simulink model "Switched_Boost_Inverter_for_Standalone_system"  (R2020a)
settings: Solver=ode45  StartTime=0.0  StopTime=1.5  RelTol=1e-3  EnableMultiTasking=on
libraries: powerlib x24, simulink x9
settings Model: Creator=SONY  LastModifiedBy=sunil
settings DataIOCC: LimitDataPoints=on  SaveFormat=Array  SignalLoggingSaveFormat=ModelDataLogs  ReturnWorkspaceOutputs=off
settings OptimizationCC: LifeSpan=inf
settings DebuggingCC: UnderspecifiedInitializationDetection=Classic  MergeDetectMultiDrivingBlocksExec=none  SolverPrmCheckMsg=warning  FcnCallInpInsideContextMsg=warning  UnconnectedInputMsg=none  UnconnectedOutputMsg=none  UnconnectedLineMsg=none  StateNameClashWarn=warning  SFUnexpectedBacktrackingDiag=warning  SFNoUnconditionalDefaultTransitionDiag=warning  SFExecutionAtInitializationDiag=none  ArithmeticOperatorsInVariantConditions=warning
settings HardwareCC: ProdBitPerPointer=32  ProdBitPerSizeT=32  ProdBitPerPtrDiffT=32  ProdLargestAtomicFloat=None  ProdIntDivRoundTo=Undefined  ProdEndianess=Unspecified  ProdWordSize=32  ProdHWDeviceType=32-bit Generic
settings ModelReferenceCC: PropagateSignalLabelsOutOfModel=off
settings SFSimCC: SimUseLocalCustomCode=off  CustomCodeUndefinedFunction=UseInterfaceOnly
settings RTWCC: RTWUseLocalCustomCode=off
settings CodeAppCC: StateflowObjectComments=on
settings GRTTargetCC: TargetLangStandard=C89/C90 (ANSI)  CombineOutputUpdateFcns=off  GRTInterface=on
settings ConfigComp: CovMetricSettings=dw  CovHtmlReporting=on  CovSaveCumulativeToWorkspaceVar=on  CovSaveSingleToWorkspaceVar=on  CovExternalEMLEnable=off
settings SimscapeCC: SimscapeNormalizeSystem=off

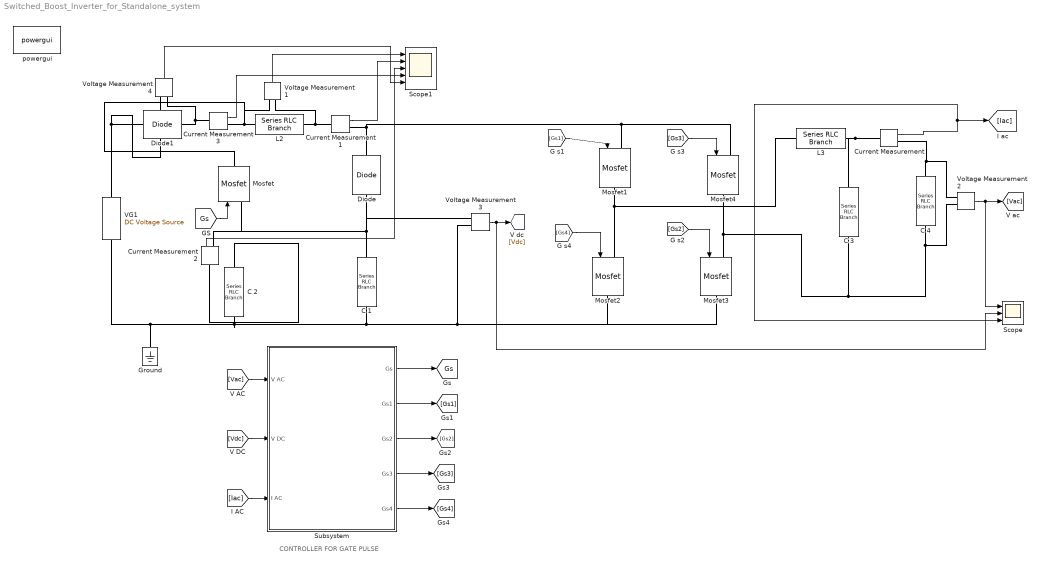
== system Switched_Boost_Inverter_for_Standalone_system ==
  note: CONTROLLER FOR GATE PULSE
  C 1 : powerlib/Elements/Series RLC Branch  LConnTagsString=__new0  RConnTagsString=__new0  BranchType=R  Resistance=70  Inductance=1e-3  SetiL0=off  InitialCurrent=0  Capacitance=1000e-6  Setx0=off  InitialVoltage=0  Measurements=None
  C 2 : powerlib/Elements/Series RLC Branch  LConnTagsString=__new0  RConnTagsString=__new0  BranchType=C  Resistance=1  Inductance=1e-3  SetiL0=off  InitialCurrent=0  Capacitance=10000e-6  Setx0=off  InitialVoltage=77  Measurements=None
  C 3 : powerlib/Elements/Series RLC Branch  LConnTagsString=__new0  RConnTagsString=__new0  BranchType=C  Resistance=1  Inductance=1e-3  SetiL0=off  InitialCurrent=0  Capacitance=.8e-3  Setx0=off  InitialVoltage=0  Measurements=None
  C 4 : powerlib/Elements/Series RLC Branch  LConnTagsString=__new0  RConnTagsString=__new0  BranchType=R  Resistance=210  Inductance=1e-3  SetiL0=off  InitialCurrent=0  Capacitance=1000e-6  Setx0=off  InitialVoltage=0  Measurements=None
  Current Measurement{,1..3} (4 alike) : powerlib/Measurements/Current Measurement  PhasorSimulation=off  OutputType=Complex  PSBequivalent=0
  Diode : powerlib/Power Electronics/Diode  Ron=0.001  Lon=0  Vf=0.8  IC=0  UseSnubber=off  Rs=inf  Cs=0  Measurements=off
  Diode1 : powerlib/Power Electronics/Diode  Ron=0.001  Lon=0  Vf=0.8  IC=0  UseSnubber=off  Rs=inf  Cs=0  Measurements=off
  Ground : powerlib/Elements/Ground  LConnTagsString=a
  L2 : powerlib/Elements/Series RLC Branch  LConnTagsString=__new0  RConnTagsString=__new0  BranchType=L  Resistance=0  Inductance=8500e-6  SetiL0=off  InitialCurrent=3  Capacitance=0  Setx0=off  InitialVoltage=0  Measurements=None
  L3 : powerlib/Elements/Series RLC Branch  LConnTagsString=__new0  RConnTagsString=__new0  BranchType=L  Resistance=0  Inductance=5e-3  SetiL0=off  InitialCurrent=0  Capacitance=0  Setx0=off  InitialVoltage=0  Measurements=None
  Mosfet{,1..4} (5 alike) : powerlib/Power Electronics/Mosfet  Ron=0.1  Lon=0  Rd=0.01  Vfd=0  IC=0  Rs=1e5  Cs=inf  Measurements=off
  Scope : Scope  NumInputPorts=3
  Scope1 : Scope  NumInputPorts=5
  Subsystem : Subsystem
  VG1 : powerlib/Electrical Sources/DC Voltage Source  Amplitude=48  Measurements=Voltage
  Voltage Measurement{1..4} (4 alike) : powerlib/Measurements/Voltage Measurement  PhasorSimulation=off  OutputType=Complex  PSBequivalent=0
  powergui : powerlib/powergui  Priority=1  SimulationMode=Discrete  SampleTime=50e-7  frequency=60  Iterations=50  frequencyindice=0  Pbase=100e6  ErrMax=1e-4  UnitsV=kV  UnitsW=MW  buscounter=0  FunctionMessages=off  echomessages=off  EnableUseOfTLC=off  CurrentSourceSwitches=off  DisableSnubberDevices=off  DisableRonSwitches=off  DisableVfSwitches=off  DisplayEquations=off  AutomaticDiscreteSolvers=off  SolverType=Tustin  Interpol=off  ExternalGateDelay=off  methode=off  Ts=0  x0status=blocks  SPID=off  SwTol=0  HookPort=off  NonlinearTolerance=1e-4  nMaxIteration=100  ContinueOnMaxIteration=off  RestoreLinks=warning  ResistiveCurrentMeasurement=off  Frange=[0:2:500]  Ylog=off  Xlog=on  ShowGrid=off  save=off  variable=ZData  structure=0  ZoomFFT=off  StartTime=0.0  cycles=1  DisplayStyle=1  fundamental=60  FreqAxis=off  MaxFrequency=1000  frequencyindicesteady=1  RmsSteady=1  display=off
  tag scope: Gs=global
  wires:
  Voltage Measurement3/1 -> Scope/2, [Vdc]
  [Gs1] -> Mosfet1/1
  [Gs4] -> Mosfet2/1
  [Gs2] -> Mosfet3/1
  Voltage Measurement2/1 -> Scope/1, [Vac]
  Subsystem/1(Gs) -> [Gs]
  Subsystem/2("Gs1 ") -> [Gs1]
  Subsystem/3(Gs2) -> [Gs2]
  Subsystem/4(Gs3) -> [Gs3]
  Subsystem/5(Gs4) -> [Gs4]
  [Vac] -> Subsystem/1(V AC)
  [Vdc] -> Subsystem/2(V DC)
  [Iac] -> Subsystem/3(I AC)
  [Gs3] -> Mosfet4/1
  Current Measurement/1 -> Scope/3, [Iac]
  Voltage Measurement1/1 -> Scope1/1
  Current Measurement1/1 -> Scope1/2
  Current Measurement2/1 -> Scope1/3
  Current Measurement3/1 -> Scope1/4
  Voltage Measurement4/1 -> Scope1/5
  [Gs] -> Mosfet/1
  connections:
  L3/LConn1 -- Mosfet2/LConn1 -- Mosfet1/RConn1
  Voltage Measurement2/LConn2 -- C 3/RConn1 -- Mosfet4/RConn1 -- Mosfet3/LConn1 -- C 4/LConn1
  VG1/LConn1 -- Ground/LConn1 -- C 1/LConn1 -- Voltage Measurement3/LConn2 -- Mosfet3/RConn1 -- Mosfet2/RConn1 -- C 2/RConn1
  C 4/RConn1 -- Current Measurement/RConn1 -- Voltage Measurement2/LConn1
  Current Measurement/LConn1 -- C 3/LConn1 -- L3/RConn1
  VG1/RConn1 -- Voltage Measurement4/LConn1 -- Diode1/LConn1
  Voltage Measurement3/LConn1 -- Diode/RConn1 -- Current Measurement2/RConn1 -- Mosfet/LConn1 -- C 1/RConn1
  Mosfet4/LConn1 -- Current Measurement1/RConn1 -- Diode/LConn1 -- Mosfet1/LConn1
  Current Measurement3/RConn1 -- Mosfet/RConn1 -- Voltage Measurement1/LConn1 -- L2/LConn1
  Current Measurement1/LConn1 -- Voltage Measurement1/LConn2 -- L2/RConn1
  C 2/LConn1 -- Current Measurement2/LConn1
  Current Measurement3/LConn1 -- Voltage Measurement4/LConn2 -- Diode1/RConn1

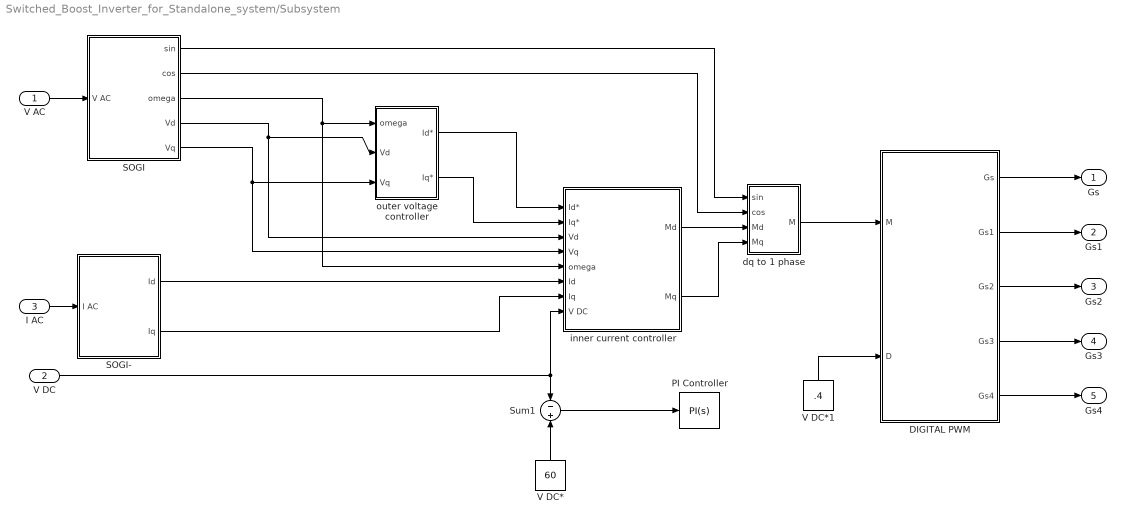
== system Switched_Boost_Inverter_for_Standalone_system/Subsystem ==
  V AC : Inport
  V DC : Inport  Port=2
  I AC : Inport  Port=3
  DIGITAL PWM : Subsystem
  PI Controller : simulink/Continuous/PID Controller  Controller=PI  Form=Parallel  TimeDomain=Continuous-time  UseExternalTs=off  SampleTime=1  IntegratorMethod=Forward Euler  FilterMethod=Forward Euler  ControllerParametersSource=internal  P=.0001  I=1  D=-0.695594942304429  UseFilter=on  N=5248.00493874348  TunerSelectOption=Transfer Function Based (PID Tuner App)  InitialConditionSource=internal  InitialConditionForIntegrator=0  InitialConditionForFilter=0  DifferentiatorICPrevScaledInput=0  ExternalReset=none  TrackingMode=off  Kt=1  LimitOutput=off  UpperSaturationLimit=inf  LowerSaturationLimit=-inf  LinearizeAsGain=off  AntiWindupMode=none  Kb=1  POutMin=[]  POutMax=[]  IOutMin=[]  IOutMax=[]  DOutMin=[]  DOutMax=[]  NOutMin=[]  NOutMax=[]  SumOutMin=[]  SumOutMax=[]  SaturationOutMin=[]  SaturationOutMax=[]  PParamMin=[]  PParamMax=[]  IParamMin=[]  IParamMax=[]  DParamMin=[]  DParamMax=[]  NParamMin=[]  NParamMax=[]  KbParamMin=[]  KbParamMax=[]  KtParamMin=[]  KtParamMax=[]  KbOutMin=[]  KbOutMax=[]  KtOutMin=[]  KtOutMax=[]  IntegratorOutMin=[]  IntegratorOutMax=[]  FilterOutMin=[]  FilterOutMax=[]  SumI1OutMin=[]  SumI1OutMax=[]  SumI2OutMin=[]  SumI2OutMax=[]  SumI3OutMin=[]  SumI3OutMax=[]  SumI4OutMin=[]  SumI4OutMax=[]  SumDOutMin=[]  SumDOutMax=[]  DifferentiatorOutMin=[]  DifferentiatorOutMax=[]  FilterDiffOutCoefMin=[]  FilterDiffOutCoefMax=[]  ReciprocalOutMin=[]  ReciprocalOutMax=[]  SumDenOutMin=[]  SumDenOutMax=[]  SumNumOutMin=[]  SumNumOutMax=[]  DivideOutMin=[]  DivideOutMax=[]  UdiffTsProdOutMin=[]  UdiffTsProdOutMax=[]  NTsProdOutMin=[]  NTsProdOutMax=[]  UintegralTsProdOutMin=[]  UintegralTsProdOutMax=[]  UngainTsProdOutMin=[]  UngainTsProdOutMax=[]  IntegratorContinuousStateAttributes=''  IntegratorStateMustResolveToSignalObject=off  IntegratorRTWStateStorageClass=Auto  FilterContinuousStateAttributes=''  FilterStateMustResolveToSignalObject=off  FilterRTWStateStorageClass=Auto  ParallelPVariant=InternalParameters  IdealPVariant=Disabled  IVariant=InternalParameters  DVariant=Disabled  IntegratorVariant=Continuous  SatVariant=Disabled  AWVariant=Passthrough  PCopyVariant=Disabled  TRVariant=Disabled  FdbkBlocksVariant=Forward  IdealPFdbkVariant=Disabled  SatFdbkVariant=Disabled  DerivativeFilterVariant=Disabled  NVariant=Disabled  NCopyVariant=Disabled_SignalSpec  FilterICVariant=Disabled  IntegratorICVariant=InternalICs  ExternalResetVariant=Disabled  TRSumVariant=Passthrough  SumFdbkVariant=Disabled  SumVariant=Sum_PI  TsampFilterVariant=InternalTs  TsampNgainVariant=Passthrough  TsampIntegralVariant=Passthrough
  SOGI : Subsystem
  SOGI- : Subsystem
  Sum1 : Sum  Inputs=-+
  V DC* : Constant  Value=60
  V DC*1 : Constant  Value=.4
  dq to 1 phase : Subsystem
  inner current controller : Subsystem
  outer voltage controller : Subsystem
  Gs : Outport  InitialOutput=0
  "Gs1 " : Outport  Port=2  InitialOutput=0
  Gs2 : Outport  Port=3  InitialOutput=0
  Gs3 : Outport  Port=4  InitialOutput=0
  Gs4 : Outport  Port=5  InitialOutput=0
  wires:
  V AC/1 -> SOGI/1(V AC)
  I AC/1 -> SOGI-/1(I AC)
  SOGI/4(Vd) -> inner current controller/3(Vd), outer voltage controller/2(Vd)
  SOGI/5(Vq) -> inner current controller/4(Vq), outer voltage controller/3(Vq)
  SOGI-/1(Id) -> inner current controller/6(Id)
  SOGI-/2(Iq) -> inner current controller/7(Iq)
  V DC/1 -> inner current controller/8(V DC), Sum1/1
  outer voltage controller/1(Id*) -> inner current controller/1(Id*)
  outer voltage controller/2(Iq*) -> inner current controller/2(Iq*)
  Sum1/1 -> PI Controller/1
  V DC*/1 -> Sum1/2
  inner current controller/1(Md) -> dq to 1 phase/3(Md)
  inner current controller/2(Mq) -> dq to 1 phase/4(Mq)
  DIGITAL PWM/1(Gs) -> Gs/1
  DIGITAL PWM/2("Gs1 ") -> "Gs1 "/1
  DIGITAL PWM/3(Gs2) -> Gs2/1
  DIGITAL PWM/4(Gs3) -> Gs3/1
  DIGITAL PWM/5(Gs4) -> Gs4/1
  SOGI/3(omega) -> inner current controller/5(omega), outer voltage controller/1(omega)
  SOGI/1(sin) -> dq to 1 phase/1(sin)
  SOGI/2(cos) -> dq to 1 phase/2(cos)
  V DC*1/1 -> DIGITAL PWM/2(D)
  dq to 1 phase/1(M) -> DIGITAL PWM/1(M)

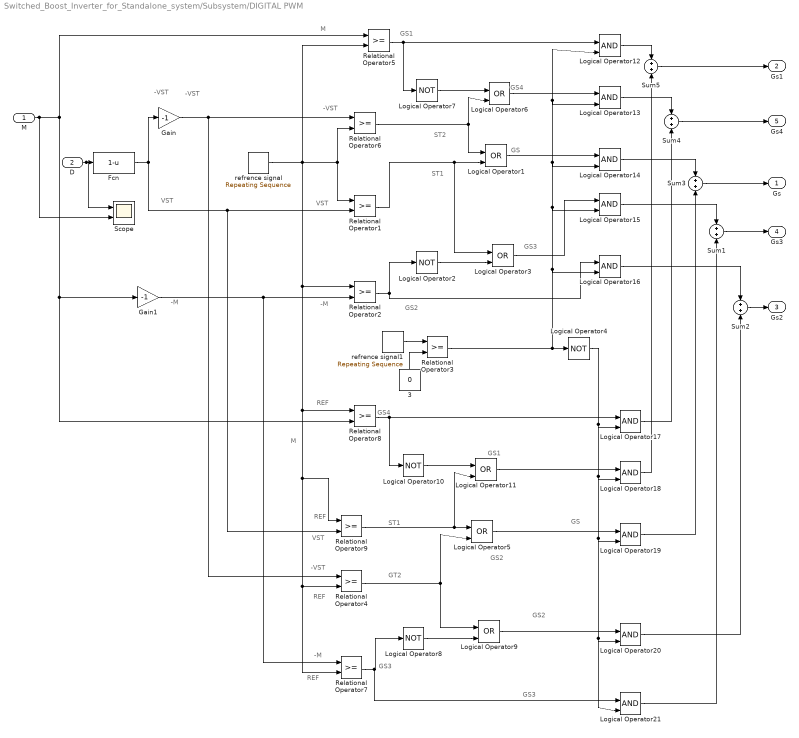
== system Switched_Boost_Inverter_for_Standalone_system/Subsystem/DIGITAL PWM ==
  note: GS3
  note: GS2
  note: GS
  note: GS2
  note: GS3
  note: GS
  note: GS4
  note: GS1
  note: -M
  note: VST
  note: -VST
  note: M
  note: GT2
  note: ST1
  note: -M
  note: -VST
  note: VST
  note: REF
  note: REF
  note: REF
  note: REF
  note: VST
  note: -VST
  note: -VST
  note: -M
  note: GS3
  note: GS2
  note: GS1
  note: GS4
  note: ST1
  note: ST2
  note: M
  M : Inport
  D : Inport  Port=2
  3 : Constant  Value=0
  Fcn : Fcn  Expr=1-u
  Gain : Gain  Gain=-1
  Gain1 : Gain  Gain=-1
  Logical Operator{1,3,5..6,9,11} (6 alike) : Logic  Operator=OR  IconShape=distinctive  AllPortsSameDT=off  OutDataTypeStr=boolean
  Logical Operator{2,4,7..8,10} (5 alike) : Logic  Operator=NOT  IconShape=distinctive  AllPortsSameDT=off  OutDataTypeStr=boolean
  Logical Operator{12..21} (10 alike) : Logic  IconShape=distinctive  AllPortsSameDT=off  OutDataTypeStr=boolean
  Relational Operator{1..9} (9 alike) : RelationalOperator  OutDataTypeStr=boolean  RndMeth=Nearest
  Scope : Scope  NumInputPorts=2
  Sum{1..5} (5 alike) : Sum
  refrence signal : simulink/Sources/Repeating Sequence  rep_seq_t="[0 .00005  .0001]"  rep_seq_y="[1 -1  1 ]"
  refrence signal1 : simulink/Sources/Repeating Sequence  rep_seq_t="[0  .01  .02]"  rep_seq_y="[1  0  -1  ]"
  Gs : Outport  InitialOutput=0
  "Gs1 " : Outport  Port=2  InitialOutput=0
  Gs2 : Outport  Port=3  InitialOutput=0
  Gs3 : Outport  Port=4  InitialOutput=0
  Gs4 : Outport  Port=5  InitialOutput=0
  wires:
  Gain/1 -> Relational Operator4/1, Relational Operator6/1
  Relational Operator5/1 -> Logical Operator7/1, Logical Operator12/1
  Logical Operator7/1 -> Logical Operator6/1
  Relational Operator6/1 -> Logical Operator1/1, Logical Operator6/2
  Relational Operator1/1 -> Logical Operator1/2, Logical Operator3/1
  Gain1/1 -> Relational Operator7/1, Relational Operator2/2
  Relational Operator2/1 -> Logical Operator2/1, Logical Operator16/1
  Logical Operator2/1 -> Logical Operator3/2
  D/1 -> Scope/1, Fcn/1
  Relational Operator8/1 -> Logical Operator17/1, Logical Operator10/1
  Logical Operator10/1 -> Logical Operator11/1
  Relational Operator9/1 -> Logical Operator11/2, Logical Operator5/1
  Relational Operator4/1 -> Logical Operator5/2, Logical Operator9/1
  Relational Operator7/1 -> Logical Operator21/1, Logical Operator8/1
  Logical Operator8/1 -> Logical Operator9/2
  Fcn/1 -> Relational Operator9/2, Relational Operator1/2, Gain/1
  refrence signal/1 -> Relational Operator8/1, Relational Operator9/1, Relational Operator4/2, Relational Operator7/2, Relational Operator2/1, Relational Operator5/2, Relational Operator1/1, Relational Operator6/2
  M/1 -> Scope/2, Relational Operator5/1, Relational Operator8/2, Gain1/1
  refrence signal1/1 -> Relational Operator3/1
  3/1 -> Relational Operator3/2
  Logical Operator4/1 -> Logical Operator20/2, Logical Operator21/2, Logical Operator19/2, Logical Operator18/2, Logical Operator17/2
  Logical Operator6/1 -> Logical Operator13/1
  Logical Operator1/1 -> Logical Operator14/1
  Logical Operator3/1 -> Logical Operator15/1
  Relational Operator3/1 -> Logical Operator16/2, Logical Operator15/2, Logical Operator14/2, Logical Operator13/2, Logical Operator12/2, Logical Operator4/1
  Logical Operator11/1 -> Logical Operator18/1
  Logical Operator5/1 -> Logical Operator19/1
  Logical Operator9/1 -> Logical Operator20/1
  Logical Operator12/1 -> Sum5/1
  Sum5/1 -> "Gs1 "/1
  Logical Operator18/1 -> Sum5/2
  Logical Operator13/1 -> Sum4/1
  Sum4/1 -> Gs4/1
  Logical Operator17/1 -> Sum4/2
  Logical Operator14/1 -> Sum3/1
  Sum3/1 -> Gs/1
  Logical Operator19/1 -> Sum3/2
  Logical Operator16/1 -> Sum2/1
  Logical Operator15/1 -> Sum1/1
  Sum1/1 -> Gs3/1
  Logical Operator21/1 -> Sum1/2
  Sum2/1 -> Gs2/1
  Logical Operator20/1 -> Sum2/2

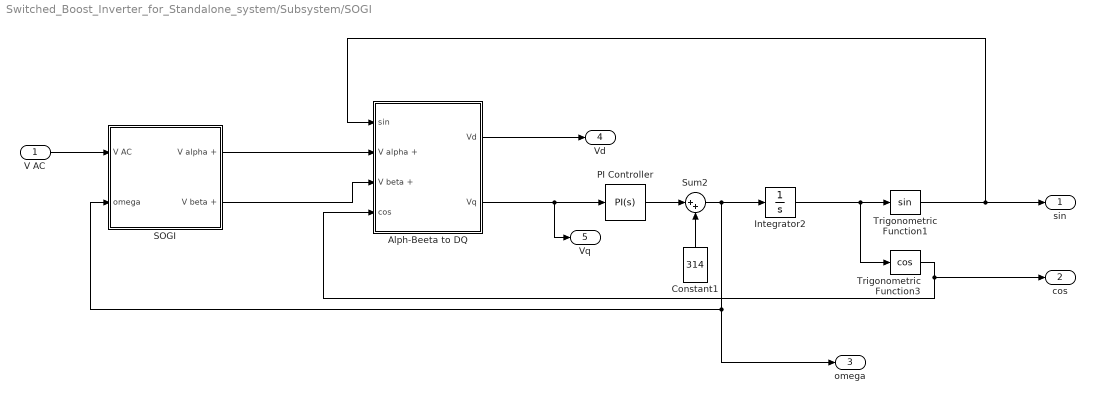
== system Switched_Boost_Inverter_for_Standalone_system/Subsystem/SOGI ==
  V AC : Inport
  Alph-Beeta to DQ : Subsystem
  Constant1 : Constant  Value=314
  Integrator2 : Integrator
  PI Controller : simulink/Continuous/PID Controller  Controller=PI  Form=Parallel  TimeDomain=Continuous-time  UseExternalTs=off  SampleTime=1  IntegratorMethod=Forward Euler  FilterMethod=Forward Euler  ControllerParametersSource=internal  P=1  I=2  D=-0.695594942304429  UseFilter=on  N=5248.00493874348  TunerSelectOption=Transfer Function Based (PID Tuner App)  InitialConditionSource=internal  InitialConditionForIntegrator=0  InitialConditionForFilter=0  DifferentiatorICPrevScaledInput=0  ExternalReset=none  TrackingMode=off  Kt=1  LimitOutput=off  UpperSaturationLimit=inf  LowerSaturationLimit=-inf  LinearizeAsGain=off  AntiWindupMode=none  Kb=1  POutMin=[]  POutMax=[]  IOutMin=[]  IOutMax=[]  DOutMin=[]  DOutMax=[]  NOutMin=[]  NOutMax=[]  SumOutMin=[]  SumOutMax=[]  SaturationOutMin=[]  SaturationOutMax=[]  PParamMin=[]  PParamMax=[]  IParamMin=[]  IParamMax=[]  DParamMin=[]  DParamMax=[]  NParamMin=[]  NParamMax=[]  KbParamMin=[]  KbParamMax=[]  KtParamMin=[]  KtParamMax=[]  KbOutMin=[]  KbOutMax=[]  KtOutMin=[]  KtOutMax=[]  IntegratorOutMin=[]  IntegratorOutMax=[]  FilterOutMin=[]  FilterOutMax=[]  SumI1OutMin=[]  SumI1OutMax=[]  SumI2OutMin=[]  SumI2OutMax=[]  SumI3OutMin=[]  SumI3OutMax=[]  SumI4OutMin=[]  SumI4OutMax=[]  SumDOutMin=[]  SumDOutMax=[]  DifferentiatorOutMin=[]  DifferentiatorOutMax=[]  FilterDiffOutCoefMin=[]  FilterDiffOutCoefMax=[]  ReciprocalOutMin=[]  ReciprocalOutMax=[]  SumDenOutMin=[]  SumDenOutMax=[]  SumNumOutMin=[]  SumNumOutMax=[]  DivideOutMin=[]  DivideOutMax=[]  UdiffTsProdOutMin=[]  UdiffTsProdOutMax=[]  NTsProdOutMin=[]  NTsProdOutMax=[]  UintegralTsProdOutMin=[]  UintegralTsProdOutMax=[]  UngainTsProdOutMin=[]  UngainTsProdOutMax=[]  IntegratorContinuousStateAttributes=''  IntegratorStateMustResolveToSignalObject=off  IntegratorRTWStateStorageClass=Auto  FilterContinuousStateAttributes=''  FilterStateMustResolveToSignalObject=off  FilterRTWStateStorageClass=Auto  ParallelPVariant=InternalParameters  IdealPVariant=Disabled  IVariant=InternalParameters  DVariant=Disabled  IntegratorVariant=Continuous  SatVariant=Disabled  AWVariant=Passthrough  PCopyVariant=Disabled  TRVariant=Disabled  FdbkBlocksVariant=Forward  IdealPFdbkVariant=Disabled  SatFdbkVariant=Disabled  DerivativeFilterVariant=Disabled  NVariant=Disabled  NCopyVariant=Disabled_SignalSpec  FilterICVariant=Disabled  IntegratorICVariant=InternalICs  ExternalResetVariant=Disabled  TRSumVariant=Passthrough  SumFdbkVariant=Disabled  SumVariant=Sum_PI  TsampFilterVariant=InternalTs  TsampNgainVariant=Passthrough  TsampIntegralVariant=Passthrough
  SOGI : Subsystem
  Sum2 : Sum  Inputs=|++
  Trigonometric Function1 : Trigonometry
  Trigonometric Function3 : Trigonometry  Operator=cos
  sin : Outport
  cos : Outport  Port=2
  omega : Outport  Port=3
  Vd : Outport  Port=4
  Vq : Outport  Port=5
  wires:
  Sum2/1 -> omega/1, SOGI/2(omega), Integrator2/1
  SOGI/1(V alpha +) -> Alph-Beeta to DQ/2(V alpha +)
  SOGI/2(V beta +) -> Alph-Beeta to DQ/3(V beta +)
  Trigonometric Function3/1 -> cos/1, Alph-Beeta to DQ/4(cos)
  Integrator2/1 -> Trigonometric Function3/1, Trigonometric Function1/1
  Alph-Beeta to DQ/1(Vd) -> Vd/1
  PI Controller/1 -> Sum2/1
  Constant1/1 -> Sum2/2
  Trigonometric Function1/1 -> Alph-Beeta to DQ/1(sin), sin/1
  Alph-Beeta to DQ/2(Vq) -> PI Controller/1, Vq/1
  V AC/1 -> SOGI/1(V AC)

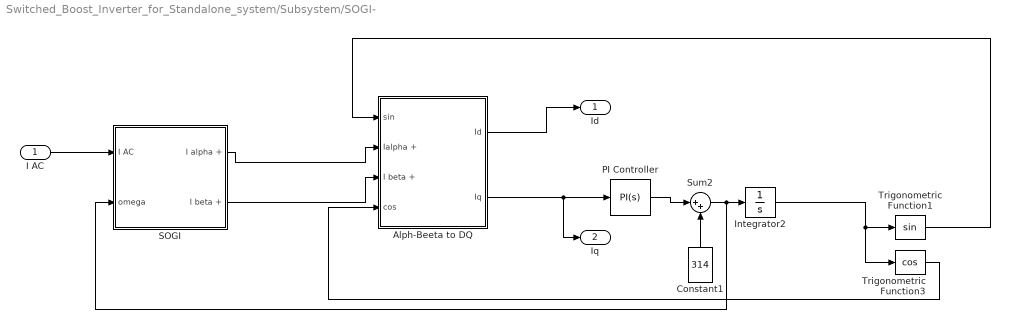
== system Switched_Boost_Inverter_for_Standalone_system/Subsystem/SOGI- ==
  I AC : Inport
  Alph-Beeta to DQ : Subsystem
  Constant1 : Constant  Value=314
  Integrator2 : Integrator
  PI Controller : simulink/Continuous/PID Controller  Controller=PI  Form=Parallel  TimeDomain=Continuous-time  UseExternalTs=off  SampleTime=1  IntegratorMethod=Forward Euler  FilterMethod=Forward Euler  ControllerParametersSource=internal  P=1  I=2  D=-0.695594942304429  UseFilter=on  N=5248.00493874348  TunerSelectOption=Transfer Function Based (PID Tuner App)  InitialConditionSource=internal  InitialConditionForIntegrator=0  InitialConditionForFilter=0  DifferentiatorICPrevScaledInput=0  ExternalReset=none  TrackingMode=off  Kt=1  LimitOutput=off  UpperSaturationLimit=inf  LowerSaturationLimit=-inf  LinearizeAsGain=off  AntiWindupMode=none  Kb=1  POutMin=[]  POutMax=[]  IOutMin=[]  IOutMax=[]  DOutMin=[]  DOutMax=[]  NOutMin=[]  NOutMax=[]  SumOutMin=[]  SumOutMax=[]  SaturationOutMin=[]  SaturationOutMax=[]  PParamMin=[]  PParamMax=[]  IParamMin=[]  IParamMax=[]  DParamMin=[]  DParamMax=[]  NParamMin=[]  NParamMax=[]  KbParamMin=[]  KbParamMax=[]  KtParamMin=[]  KtParamMax=[]  KbOutMin=[]  KbOutMax=[]  KtOutMin=[]  KtOutMax=[]  IntegratorOutMin=[]  IntegratorOutMax=[]  FilterOutMin=[]  FilterOutMax=[]  SumI1OutMin=[]  SumI1OutMax=[]  SumI2OutMin=[]  SumI2OutMax=[]  SumI3OutMin=[]  SumI3OutMax=[]  SumI4OutMin=[]  SumI4OutMax=[]  SumDOutMin=[]  SumDOutMax=[]  DifferentiatorOutMin=[]  DifferentiatorOutMax=[]  FilterDiffOutCoefMin=[]  FilterDiffOutCoefMax=[]  ReciprocalOutMin=[]  ReciprocalOutMax=[]  SumDenOutMin=[]  SumDenOutMax=[]  SumNumOutMin=[]  SumNumOutMax=[]  DivideOutMin=[]  DivideOutMax=[]  UdiffTsProdOutMin=[]  UdiffTsProdOutMax=[]  NTsProdOutMin=[]  NTsProdOutMax=[]  UintegralTsProdOutMin=[]  UintegralTsProdOutMax=[]  UngainTsProdOutMin=[]  UngainTsProdOutMax=[]  IntegratorContinuousStateAttributes=''  IntegratorStateMustResolveToSignalObject=off  IntegratorRTWStateStorageClass=Auto  FilterContinuousStateAttributes=''  FilterStateMustResolveToSignalObject=off  FilterRTWStateStorageClass=Auto  ParallelPVariant=InternalParameters  IdealPVariant=Disabled  IVariant=InternalParameters  DVariant=Disabled  IntegratorVariant=Continuous  SatVariant=Disabled  AWVariant=Passthrough  PCopyVariant=Disabled  TRVariant=Disabled  FdbkBlocksVariant=Forward  IdealPFdbkVariant=Disabled  SatFdbkVariant=Disabled  DerivativeFilterVariant=Disabled  NVariant=Disabled  NCopyVariant=Disabled_SignalSpec  FilterICVariant=Disabled  IntegratorICVariant=InternalICs  ExternalResetVariant=Disabled  TRSumVariant=Passthrough  SumFdbkVariant=Disabled  SumVariant=Sum_PI  TsampFilterVariant=InternalTs  TsampNgainVariant=Passthrough  TsampIntegralVariant=Passthrough
  SOGI : Subsystem
  Sum2 : Sum  Inputs=|++
  Trigonometric Function1 : Trigonometry
  Trigonometric Function3 : Trigonometry  Operator=cos
  Id : Outport
  Iq : Outport  Port=2
  wires:
  Sum2/1 -> SOGI/2(omega), Integrator2/1
  SOGI/1(I alpha +) -> Alph-Beeta to DQ/2(Ialpha +)
  SOGI/2(I beta +) -> Alph-Beeta to DQ/3(I beta +)
  Trigonometric Function3/1 -> Alph-Beeta to DQ/4(cos)
  Integrator2/1 -> Trigonometric Function1/1, Trigonometric Function3/1
  Alph-Beeta to DQ/1(Id) -> Id/1
  PI Controller/1 -> Sum2/1
  Constant1/1 -> Sum2/2
  Trigonometric Function1/1 -> Alph-Beeta to DQ/1(sin)
  Alph-Beeta to DQ/2(Iq) -> Iq/1, PI Controller/1
  I AC/1 -> SOGI/1(I AC)

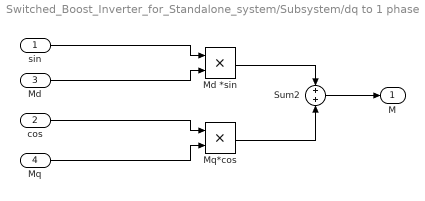
== system Switched_Boost_Inverter_for_Standalone_system/Subsystem/dq to 1 phase ==
  sin : Inport
  cos : Inport  Port=2
  Md : Inport  Port=3
  Mq : Inport  Port=4
  Md *sin : Product  Inputs=**
  Mq*cos : Product  Inputs=**
  Sum2 : Sum
  M : Outport  InitialOutput=0
  wires:
  Md/1 -> Md *sin/2
  cos/1 -> Mq*cos/1
  Mq*cos/1 -> Sum2/2
  Sum2/1 -> M/1
  Mq/1 -> Mq*cos/2
  Md *sin/1 -> Sum2/1
  sin/1 -> Md *sin/1

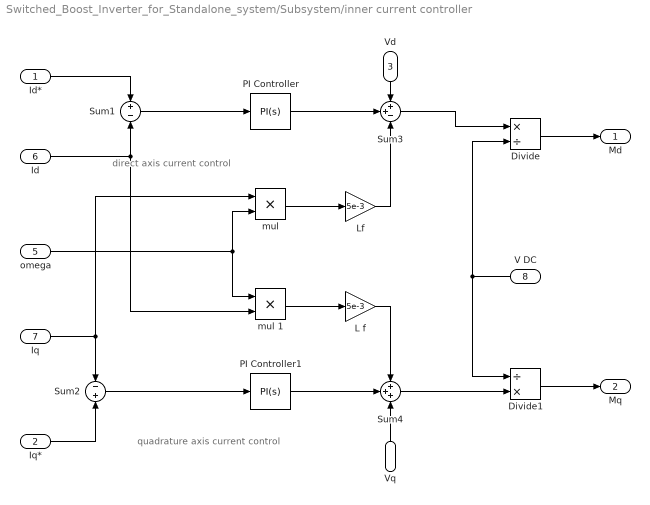
== system Switched_Boost_Inverter_for_Standalone_system/Subsystem/inner current controller ==
  note: quadrature axis current control
  note: direct axis current control
  Id* : Inport
  Iq* : Inport  Port=2
  Vd : Inport  Port=3
  Vq : Inport  Port=4
  omega : Inport  Port=5
  Id : Inport  Port=6
  Iq : Inport  Port=7
  V DC : Inport  Port=8
  Divide : Product  Inputs=*/
  Divide1 : Product  Inputs=/*
  L f : Gain  Gain=5e-3
  Lf : Gain  Gain=5e-3
  PI Controller : simulink/Continuous/PID Controller  Controller=PI  Form=Parallel  TimeDomain=Continuous-time  UseExternalTs=off  SampleTime=1  IntegratorMethod=Forward Euler  FilterMethod=Forward Euler  ControllerParametersSource=internal  P=.01  I=.09  D=-0.695594942304429  UseFilter=on  N=5248.00493874348  TunerSelectOption=Transfer Function Based (PID Tuner App)  InitialConditionSource=internal  InitialConditionForIntegrator=0  InitialConditionForFilter=0  DifferentiatorICPrevScaledInput=0  ExternalReset=none  TrackingMode=off  Kt=1  LimitOutput=off  UpperSaturationLimit=inf  LowerSaturationLimit=-inf  LinearizeAsGain=off  AntiWindupMode=none  Kb=1  POutMin=[]  POutMax=[]  IOutMin=[]  IOutMax=[]  DOutMin=[]  DOutMax=[]  NOutMin=[]  NOutMax=[]  SumOutMin=[]  SumOutMax=[]  SaturationOutMin=[]  SaturationOutMax=[]  PParamMin=[]  PParamMax=[]  IParamMin=[]  IParamMax=[]  DParamMin=[]  DParamMax=[]  NParamMin=[]  NParamMax=[]  KbParamMin=[]  KbParamMax=[]  KtParamMin=[]  KtParamMax=[]  KbOutMin=[]  KbOutMax=[]  KtOutMin=[]  KtOutMax=[]  IntegratorOutMin=[]  IntegratorOutMax=[]  FilterOutMin=[]  FilterOutMax=[]  SumI1OutMin=[]  SumI1OutMax=[]  SumI2OutMin=[]  SumI2OutMax=[]  SumI3OutMin=[]  SumI3OutMax=[]  SumI4OutMin=[]  SumI4OutMax=[]  SumDOutMin=[]  SumDOutMax=[]  DifferentiatorOutMin=[]  DifferentiatorOutMax=[]  FilterDiffOutCoefMin=[]  FilterDiffOutCoefMax=[]  ReciprocalOutMin=[]  ReciprocalOutMax=[]  SumDenOutMin=[]  SumDenOutMax=[]  SumNumOutMin=[]  SumNumOutMax=[]  DivideOutMin=[]  DivideOutMax=[]  UdiffTsProdOutMin=[]  UdiffTsProdOutMax=[]  NTsProdOutMin=[]  NTsProdOutMax=[]  UintegralTsProdOutMin=[]  UintegralTsProdOutMax=[]  UngainTsProdOutMin=[]  UngainTsProdOutMax=[]  IntegratorContinuousStateAttributes=''  IntegratorStateMustResolveToSignalObject=off  IntegratorRTWStateStorageClass=Auto  FilterContinuousStateAttributes=''  FilterStateMustResolveToSignalObject=off  FilterRTWStateStorageClass=Auto  ParallelPVariant=InternalParameters  IdealPVariant=Disabled  IVariant=InternalParameters  DVariant=Disabled  IntegratorVariant=Continuous  SatVariant=Disabled  AWVariant=Passthrough  PCopyVariant=Disabled  TRVariant=Disabled  FdbkBlocksVariant=Forward  IdealPFdbkVariant=Disabled  SatFdbkVariant=Disabled  DerivativeFilterVariant=Disabled  NVariant=Disabled  NCopyVariant=Disabled_SignalSpec  FilterICVariant=Disabled  IntegratorICVariant=InternalICs  ExternalResetVariant=Disabled  TRSumVariant=Passthrough  SumFdbkVariant=Disabled  SumVariant=Sum_PI  TsampFilterVariant=InternalTs  TsampNgainVariant=Passthrough  TsampIntegralVariant=Passthrough
  PI Controller1 : simulink/Continuous/PID Controller  Controller=PI  Form=Parallel  TimeDomain=Continuous-time  UseExternalTs=off  SampleTime=1  IntegratorMethod=Forward Euler  FilterMethod=Forward Euler  ControllerParametersSource=internal  P=.01  I=.09  D=-0.695594942304429  UseFilter=on  N=5248.00493874348  TunerSelectOption=Transfer Function Based (PID Tuner App)  InitialConditionSource=internal  InitialConditionForIntegrator=0  InitialConditionForFilter=0  DifferentiatorICPrevScaledInput=0  ExternalReset=none  TrackingMode=off  Kt=1  LimitOutput=off  UpperSaturationLimit=inf  LowerSaturationLimit=-inf  LinearizeAsGain=off  AntiWindupMode=none  Kb=1  POutMin=[]  POutMax=[]  IOutMin=[]  IOutMax=[]  DOutMin=[]  DOutMax=[]  NOutMin=[]  NOutMax=[]  SumOutMin=[]  SumOutMax=[]  SaturationOutMin=[]  SaturationOutMax=[]  PParamMin=[]  PParamMax=[]  IParamMin=[]  IParamMax=[]  DParamMin=[]  DParamMax=[]  NParamMin=[]  NParamMax=[]  KbParamMin=[]  KbParamMax=[]  KtParamMin=[]  KtParamMax=[]  KbOutMin=[]  KbOutMax=[]  KtOutMin=[]  KtOutMax=[]  IntegratorOutMin=[]  IntegratorOutMax=[]  FilterOutMin=[]  FilterOutMax=[]  SumI1OutMin=[]  SumI1OutMax=[]  SumI2OutMin=[]  SumI2OutMax=[]  SumI3OutMin=[]  SumI3OutMax=[]  SumI4OutMin=[]  SumI4OutMax=[]  SumDOutMin=[]  SumDOutMax=[]  DifferentiatorOutMin=[]  DifferentiatorOutMax=[]  FilterDiffOutCoefMin=[]  FilterDiffOutCoefMax=[]  ReciprocalOutMin=[]  ReciprocalOutMax=[]  SumDenOutMin=[]  SumDenOutMax=[]  SumNumOutMin=[]  SumNumOutMax=[]  DivideOutMin=[]  DivideOutMax=[]  UdiffTsProdOutMin=[]  UdiffTsProdOutMax=[]  NTsProdOutMin=[]  NTsProdOutMax=[]  UintegralTsProdOutMin=[]  UintegralTsProdOutMax=[]  UngainTsProdOutMin=[]  UngainTsProdOutMax=[]  IntegratorContinuousStateAttributes=''  IntegratorStateMustResolveToSignalObject=off  IntegratorRTWStateStorageClass=Auto  FilterContinuousStateAttributes=''  FilterStateMustResolveToSignalObject=off  FilterRTWStateStorageClass=Auto  ParallelPVariant=InternalParameters  IdealPVariant=Disabled  IVariant=InternalParameters  DVariant=Disabled  IntegratorVariant=Continuous  SatVariant=Disabled  AWVariant=Passthrough  PCopyVariant=Disabled  TRVariant=Disabled  FdbkBlocksVariant=Forward  IdealPFdbkVariant=Disabled  SatFdbkVariant=Disabled  DerivativeFilterVariant=Disabled  NVariant=Disabled  NCopyVariant=Disabled_SignalSpec  FilterICVariant=Disabled  IntegratorICVariant=InternalICs  ExternalResetVariant=Disabled  TRSumVariant=Passthrough  SumFdbkVariant=Disabled  SumVariant=Sum_PI  TsampFilterVariant=InternalTs  TsampNgainVariant=Passthrough  TsampIntegralVariant=Passthrough
  Sum1 : Sum  Inputs=+-
  Sum2 : Sum  Inputs=-+
  Sum3 : Sum  Inputs=++-
  Sum4 : Sum  Inputs=+++
  "mul " : Product  Inputs=**
  mul 1 : Product  Inputs=**
  Md : Outport
  Mq : Outport  Port=2
  wires:
  Id/1 -> Sum1/2, mul 1/2
  Sum1/1 -> PI Controller/1
  Sum2/1 -> PI Controller1/1
  Iq/1 -> "mul "/1, Sum2/1
  Id*/1 -> Sum1/1
  Iq*/1 -> Sum2/2
  PI Controller/1 -> Sum3/2
  Vd/1 -> Sum3/1
  Vq/1 -> Sum4/3
  Sum3/1 -> Divide/1
  Sum4/1 -> Divide1/2
  V DC/1 -> Divide/2, Divide1/1
  Divide/1 -> Md/1
  Divide1/1 -> Mq/1
  PI Controller1/1 -> Sum4/2
  "mul "/1 -> Lf/1
  Lf/1 -> Sum3/3
  L f/1 -> Sum4/1
  mul 1/1 -> L f/1
  omega/1 -> "mul "/2, mul 1/1

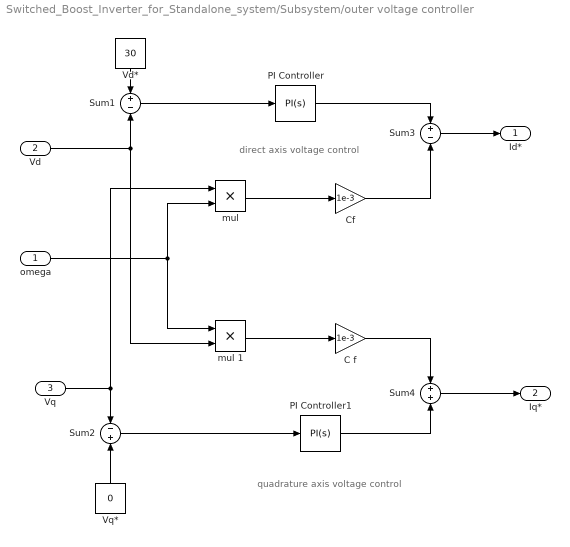
== system Switched_Boost_Inverter_for_Standalone_system/Subsystem/outer voltage controller ==
  note: quadrature axis voltage control
  note: direct axis voltage control
  omega : Inport
  Vd : Inport  Port=2
  Vq : Inport  Port=3
  C f : Gain  Gain=1e-3
  Cf : Gain  Gain=1e-3
  PI Controller : simulink/Continuous/PID Controller  Controller=PI  Form=Parallel  TimeDomain=Continuous-time  UseExternalTs=off  SampleTime=1  IntegratorMethod=Forward Euler  FilterMethod=Forward Euler  ControllerParametersSource=internal  P=67  I=100  D=-0.695594942304429  UseFilter=on  N=5248.00493874348  TunerSelectOption=Transfer Function Based (PID Tuner App)  InitialConditionSource=internal  InitialConditionForIntegrator=0  InitialConditionForFilter=0  DifferentiatorICPrevScaledInput=0  ExternalReset=none  TrackingMode=off  Kt=1  LimitOutput=off  UpperSaturationLimit=inf  LowerSaturationLimit=-inf  LinearizeAsGain=off  AntiWindupMode=none  Kb=1  POutMin=[]  POutMax=[]  IOutMin=[]  IOutMax=[]  DOutMin=[]  DOutMax=[]  NOutMin=[]  NOutMax=[]  SumOutMin=[]  SumOutMax=[]  SaturationOutMin=[]  SaturationOutMax=[]  PParamMin=[]  PParamMax=[]  IParamMin=[]  IParamMax=[]  DParamMin=[]  DParamMax=[]  NParamMin=[]  NParamMax=[]  KbParamMin=[]  KbParamMax=[]  KtParamMin=[]  KtParamMax=[]  KbOutMin=[]  KbOutMax=[]  KtOutMin=[]  KtOutMax=[]  IntegratorOutMin=[]  IntegratorOutMax=[]  FilterOutMin=[]  FilterOutMax=[]  SumI1OutMin=[]  SumI1OutMax=[]  SumI2OutMin=[]  SumI2OutMax=[]  SumI3OutMin=[]  SumI3OutMax=[]  SumI4OutMin=[]  SumI4OutMax=[]  SumDOutMin=[]  SumDOutMax=[]  DifferentiatorOutMin=[]  DifferentiatorOutMax=[]  FilterDiffOutCoefMin=[]  FilterDiffOutCoefMax=[]  ReciprocalOutMin=[]  ReciprocalOutMax=[]  SumDenOutMin=[]  SumDenOutMax=[]  SumNumOutMin=[]  SumNumOutMax=[]  DivideOutMin=[]  DivideOutMax=[]  UdiffTsProdOutMin=[]  UdiffTsProdOutMax=[]  NTsProdOutMin=[]  NTsProdOutMax=[]  UintegralTsProdOutMin=[]  UintegralTsProdOutMax=[]  UngainTsProdOutMin=[]  UngainTsProdOutMax=[]  IntegratorContinuousStateAttributes=''  IntegratorStateMustResolveToSignalObject=off  IntegratorRTWStateStorageClass=Auto  FilterContinuousStateAttributes=''  FilterStateMustResolveToSignalObject=off  FilterRTWStateStorageClass=Auto  ParallelPVariant=InternalParameters  IdealPVariant=Disabled  IVariant=InternalParameters  DVariant=Disabled  IntegratorVariant=Continuous  SatVariant=Disabled  AWVariant=Passthrough  PCopyVariant=Disabled  TRVariant=Disabled  FdbkBlocksVariant=Forward  IdealPFdbkVariant=Disabled  SatFdbkVariant=Disabled  DerivativeFilterVariant=Disabled  NVariant=Disabled  NCopyVariant=Disabled_SignalSpec  FilterICVariant=Disabled  IntegratorICVariant=InternalICs  ExternalResetVariant=Disabled  TRSumVariant=Passthrough  SumFdbkVariant=Disabled  SumVariant=Sum_PI  TsampFilterVariant=InternalTs  TsampNgainVariant=Passthrough  TsampIntegralVariant=Passthrough
  PI Controller1 : simulink/Continuous/PID Controller  Controller=PI  Form=Parallel  TimeDomain=Continuous-time  UseExternalTs=off  SampleTime=1  IntegratorMethod=Forward Euler  FilterMethod=Forward Euler  ControllerParametersSource=internal  P=67  I=100  D=-0.695594942304429  UseFilter=on  N=5248.00493874348  TunerSelectOption=Transfer Function Based (PID Tuner App)  InitialConditionSource=internal  InitialConditionForIntegrator=0  InitialConditionForFilter=0  DifferentiatorICPrevScaledInput=0  ExternalReset=none  TrackingMode=off  Kt=1  LimitOutput=off  UpperSaturationLimit=inf  LowerSaturationLimit=-inf  LinearizeAsGain=off  AntiWindupMode=none  Kb=1  POutMin=[]  POutMax=[]  IOutMin=[]  IOutMax=[]  DOutMin=[]  DOutMax=[]  NOutMin=[]  NOutMax=[]  SumOutMin=[]  SumOutMax=[]  SaturationOutMin=[]  SaturationOutMax=[]  PParamMin=[]  PParamMax=[]  IParamMin=[]  IParamMax=[]  DParamMin=[]  DParamMax=[]  NParamMin=[]  NParamMax=[]  KbParamMin=[]  KbParamMax=[]  KtParamMin=[]  KtParamMax=[]  KbOutMin=[]  KbOutMax=[]  KtOutMin=[]  KtOutMax=[]  IntegratorOutMin=[]  IntegratorOutMax=[]  FilterOutMin=[]  FilterOutMax=[]  SumI1OutMin=[]  SumI1OutMax=[]  SumI2OutMin=[]  SumI2OutMax=[]  SumI3OutMin=[]  SumI3OutMax=[]  SumI4OutMin=[]  SumI4OutMax=[]  SumDOutMin=[]  SumDOutMax=[]  DifferentiatorOutMin=[]  DifferentiatorOutMax=[]  FilterDiffOutCoefMin=[]  FilterDiffOutCoefMax=[]  ReciprocalOutMin=[]  ReciprocalOutMax=[]  SumDenOutMin=[]  SumDenOutMax=[]  SumNumOutMin=[]  SumNumOutMax=[]  DivideOutMin=[]  DivideOutMax=[]  UdiffTsProdOutMin=[]  UdiffTsProdOutMax=[]  NTsProdOutMin=[]  NTsProdOutMax=[]  UintegralTsProdOutMin=[]  UintegralTsProdOutMax=[]  UngainTsProdOutMin=[]  UngainTsProdOutMax=[]  IntegratorContinuousStateAttributes=''  IntegratorStateMustResolveToSignalObject=off  IntegratorRTWStateStorageClass=Auto  FilterContinuousStateAttributes=''  FilterStateMustResolveToSignalObject=off  FilterRTWStateStorageClass=Auto  ParallelPVariant=InternalParameters  IdealPVariant=Disabled  IVariant=InternalParameters  DVariant=Disabled  IntegratorVariant=Continuous  SatVariant=Disabled  AWVariant=Passthrough  PCopyVariant=Disabled  TRVariant=Disabled  FdbkBlocksVariant=Forward  IdealPFdbkVariant=Disabled  SatFdbkVariant=Disabled  DerivativeFilterVariant=Disabled  NVariant=Disabled  NCopyVariant=Disabled_SignalSpec  FilterICVariant=Disabled  IntegratorICVariant=InternalICs  ExternalResetVariant=Disabled  TRSumVariant=Passthrough  SumFdbkVariant=Disabled  SumVariant=Sum_PI  TsampFilterVariant=InternalTs  TsampNgainVariant=Passthrough  TsampIntegralVariant=Passthrough
  Sum1 : Sum  Inputs=+-
  Sum2 : Sum  Inputs=-+
  Sum3 : Sum  Inputs=+-
  Sum4 : Sum
  Vd* : Constant  Value=30
  Vq* : Constant  Value=0
  "mul " : Product  Inputs=**
  mul 1 : Product  Inputs=**
  Id* : Outport
  Iq* : Outport  Port=2
  wires:
  Vd/1 -> mul 1/2, Sum1/2
  Vd*/1 -> Sum1/1
  Sum1/1 -> PI Controller/1
  Sum2/1 -> PI Controller1/1
  Vq*/1 -> Sum2/2
  Vq/1 -> "mul "/1, Sum2/1
  Sum3/1 -> Id*/1
  Sum4/1 -> Iq*/1
  Cf/1 -> Sum3/2
  C f/1 -> Sum4/1
  "mul "/1 -> Cf/1
  mul 1/1 -> C f/1
  omega/1 -> mul 1/1, "mul "/2
  PI Controller/1 -> Sum3/1
  PI Controller1/1 -> Sum4/2

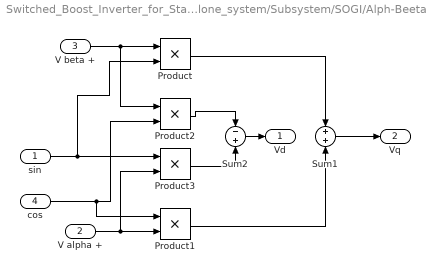
== system Switched_Boost_Inverter_for_Standalone_system/Subsystem/SOGI/Alph-Beeta to DQ ==
  sin : Inport
  V alpha + : Inport  Port=2
  V beta + : Inport  Port=3
  cos : Inport  Port=4
  Product{,1..3} (4 alike) : Product  RndMeth=Zero
  Sum1 : Sum
  Sum2 : Sum  Inputs=-+
  Vd : Outport
  Vq : Outport  Port=2
  wires:
  V beta +/1 -> Product/1, Product2/1
  V alpha +/1 -> Product3/2, Product1/2
  Product/1 -> Sum1/1
  Product1/1 -> Sum1/2
  Product2/1 -> Sum2/1
  Product3/1 -> Sum2/2
  Sum1/1 -> Vq/1
  Sum2/1 -> Vd/1
  sin/1 -> Product/2, Product3/1
  cos/1 -> Product2/2, Product1/1

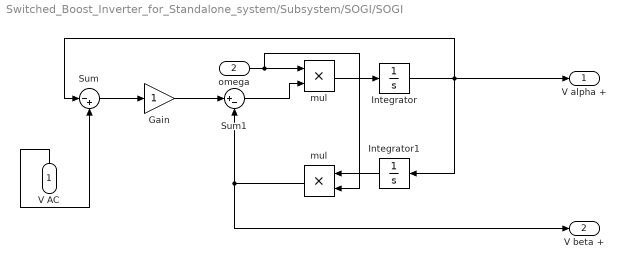
== system Switched_Boost_Inverter_for_Standalone_system/Subsystem/SOGI/SOGI ==
  V AC : Inport
  omega : Inport  Port=2
  Gain : Gain
  Integrator : Integrator
  Integrator1 : Integrator
  Sum : Sum  Inputs=|-+
  Sum1 : Sum  Inputs=|+-
  mul : Product  Inputs=**
  "mul " : Product  Inputs=**
  V alpha + : Outport
  V beta + : Outport  Port=2
  wires:
  "mul "/1 -> V beta +/1, Sum1/2
  Integrator/1 -> V alpha +/1, Integrator1/1, Sum/1
  mul/1 -> Integrator/1
  Sum1/1 -> mul/2
  Gain/1 -> Sum1/1
  Sum/1 -> Gain/1
  omega/1 -> mul/1, "mul "/2
  Integrator1/1 -> "mul "/1
  V AC/1 -> Sum/2

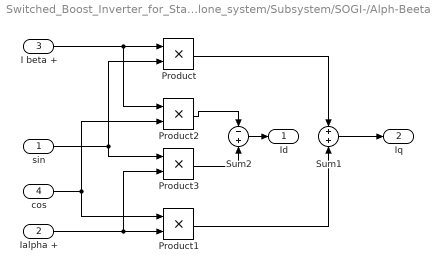
== system Switched_Boost_Inverter_for_Standalone_system/Subsystem/SOGI-/Alph-Beeta to DQ ==
  sin : Inport
  Ialpha + : Inport  Port=2
  I beta + : Inport  Port=3
  cos : Inport  Port=4
  Product{,1..3} (4 alike) : Product  RndMeth=Zero
  Sum1 : Sum
  Sum2 : Sum  Inputs=-+
  Id : Outport
  Iq : Outport  Port=2
  wires:
  I beta +/1 -> Product/1, Product2/1
  Ialpha +/1 -> Product3/2, Product1/2
  Product/1 -> Sum1/1
  Product1/1 -> Sum1/2
  Product2/1 -> Sum2/1
  Product3/1 -> Sum2/2
  Sum1/1 -> Iq/1
  Sum2/1 -> Id/1
  sin/1 -> Product3/1, Product/2
  cos/1 -> Product1/1, Product2/2

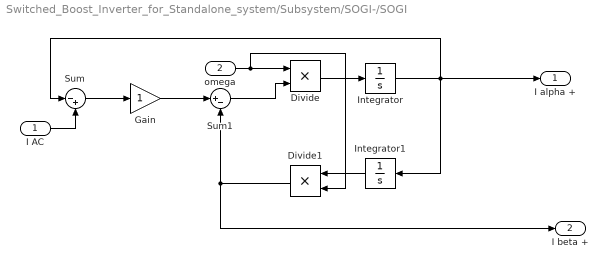
== system Switched_Boost_Inverter_for_Standalone_system/Subsystem/SOGI-/SOGI ==
  I AC : Inport
  omega : Inport  Port=2
  Divide : Product  Inputs=**
  Divide1 : Product  Inputs=**
  Gain : Gain
  Integrator : Integrator
  Integrator1 : Integrator
  Sum : Sum  Inputs=|-+
  Sum1 : Sum  Inputs=|+-
  I alpha + : Outport
  I beta + : Outport  Port=2
  wires:
  Divide1/1 -> I beta +/1, Sum1/2
  Integrator/1 -> I alpha +/1, Integrator1/1, Sum/1
  Divide/1 -> Integrator/1
  Sum1/1 -> Divide/2
  Gain/1 -> Sum1/1
  Sum/1 -> Gain/1
  omega/1 -> Divide/1, Divide1/2
  Integrator1/1 -> Divide1/1
  I AC/1 -> Sum/2
